simulink model "bergman"  (R2021a)
settings: Solver=FixedStepAuto  StartTime=0.0  StopTime=1440  FixedStep=Ts  RelTol=1e-3
values from neighbouring files (symbols this model uses):
  Ag = 0.95    [afterGA.m]    (also in identik.m; lakaka.m; surove.m)
  Gb = 153    [afterGA.m]    (also in bergmanGA.m = glucose(1); cv3.m = glucose(1); cv3a.m = glucose(1); cv4_bergman.m)
  Ib = 12.3165    [afterGA.m]    (also in bergmanGA.m = insuline(1); cv3.m = insuline(1); cv3a.m = insuline(1); cv4.m)
  kI = 0.1645    [afterGA.m]    (also in cv4.m = Best(2); cv4GA.m = Best(2); cv4_bergman.m; cv4_bergmanGA.m)
  p2 = 0.0106    [afterGA.m]    (also in cv3.m = 0.032736; cv3a.m = 0.063098; cv4_bergman.m = Best(2) / 10; cv4_bergmanGA.m = Best(2) / 10)
  S1b = 1.2528e4    (= 12528)    [afterGA.m]    (also in cv4.m; cv4GA.m; cv4_bergman.m; cv4_bergmanGA.m)
  S2b = S1b    (= 12528)    [afterGA.m]    (also in cv4.m; cv4GA.m; cv4_bergman.m; cv4_bergmanGA.m)
  Sg = 0.032    [afterGA.m]    (also in cv3.m = 0.030031; cv3a.m = 3.3574e-10; cv4_bergman.m = 0; cv4_bergmanGA.m = 0)
  Si = 0.00159    [afterGA.m]    (also in cv3.m = 1.0278e-13; cv3a.m = 0.00089844; cv4_bergman.m = Best(1) / 10; cv4_bergmanGA.m = Best(1) / 10)
  Td = 33.474    [afterGA.m]    (also in identified.mat = 40.284; identified1.mat = 33.5; lakaka.m; surove.m)
  TI = 44.55    [afterGA.m]    (also in cv4.m = Best(1); cv4GA.m = Best(1); cv4_bergman.m; cv4_bergmanGA.m)
  Vg = 1.467    [afterGA.m]    (also in cv4_bergman.m; cv4_bergmanGA.m; identik.m; lakaka.m)
  VI = 138.8    [afterGA.m]    (also in cv4.m = Best(3); cv4GA.m = Best(3); cv4_bergman.m; cv4_bergmanGA.m)
settings Model: Creator=marko  LastModifiedBy=marko

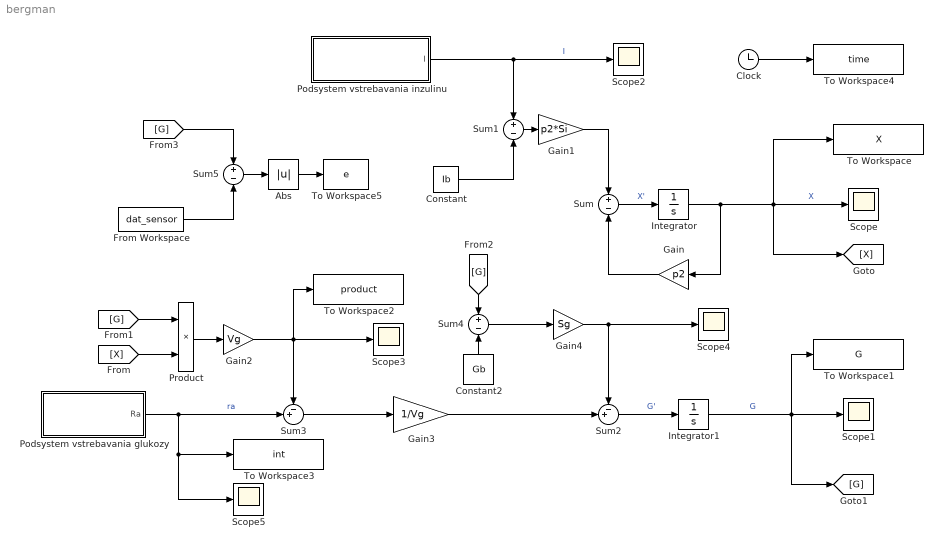
== system bergman ==
  Abs : Abs
  Clock : Clock
  Constant : Constant  Value=Ib
  Constant2 : Constant  Value=Gb
  From Workspace : FromWorkspace  VariableName=dat_sensor  Interpolate=off  OutputAfterFinalValue=Holding final value
  Gain : Gain  Gain=p2
  Gain1 : Gain  Gain=p2*Si
  Gain2 : Gain  Gain=Vg
  Gain3 : Gain  Gain=1/Vg
  Gain4 : Gain  Gain=Sg
  Integrator : Integrator
  Integrator1 : Integrator  InitialCondition=Gb
  Podsystem vstrebavania glukozy : Subsystem
  Podsystem vstrebavania inzulinu : Subsystem
  Product : Product
  Scope{,1..5} (6 alike) : Scope
  Sum{,1,4..5} (4 alike) : Sum  Inputs=+|-
  Sum2 : Sum  Inputs=-+|
  Sum3 : Sum  Inputs=-+|
  To Workspace : ToWorkspace  VariableName=X  SampleTime=-1
  To Workspace1 : ToWorkspace  VariableName=G  SampleTime=-1
  To Workspace2 : ToWorkspace  VariableName=product  SampleTime=-1
  To Workspace3 : ToWorkspace  VariableName=int  SampleTime=-1
  To Workspace4 : ToWorkspace  VariableName=time  SampleTime=-1
  To Workspace5 : ToWorkspace  VariableName=e  SampleTime=-1
  wires:
  Integrator/1 -> To Workspace/1, [X], Scope/1, Gain/1  "X"
  Gain/1 -> Sum/2
  Sum/1 -> Integrator/1  "X'"
  Constant/1 -> Sum1/2
  Sum1/1 -> Gain1/1
  Gain1/1 -> Sum/1
  Integrator1/1 -> Scope1/1, [G], To Workspace1/1  "G"
  Sum2/1 -> Integrator1/1  "G'"
  Podsystem vstrebavania inzulinu/1(I) -> Sum1/1, Scope2/1  "I"
  Podsystem vstrebavania glukozy/1(Ra) -> Scope5/1, To Workspace3/1, Sum3/2  "ra"
  Sum3/1 -> Gain3/1
  [G] -> Product/1
  [X] -> Product/2
  Product/1 -> Gain2/1
  Gain2/1 -> Scope3/1, To Workspace2/1, Sum3/1
  Gain3/1 -> Sum2/2
  [G] -> Sum4/1
  Constant2/1 -> Sum4/2
  Sum4/1 -> Gain4/1
  Gain4/1 -> Scope4/1, Sum2/1
  Clock/1 -> To Workspace4/1
  [G] -> Sum5/1
  From Workspace/1 -> Sum5/2
  Sum5/1 -> Abs/1
  Abs/1 -> To Workspace5/1

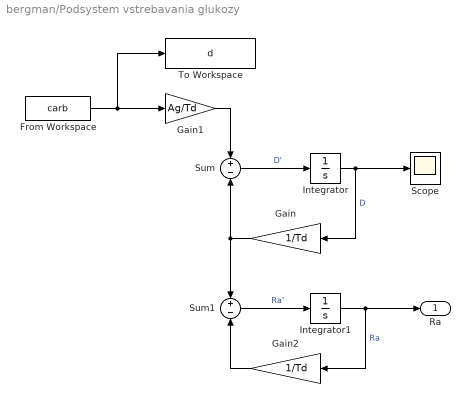
== system bergman/Podsystem vstrebavania glukozy ==
  From Workspace : FromWorkspace  VariableName=carb  Interpolate=off  OutputAfterFinalValue=Setting to zero
  Gain : Gain  Gain=1/Td
  Gain1 : Gain  Gain=Ag/Td
  Gain2 : Gain  Gain=1/Td
  Integrator : Integrator
  Integrator1 : Integrator
  Scope : Scope
  Sum : Sum  Inputs=+|-
  Sum1 : Sum  Inputs=+|-
  To Workspace : ToWorkspace  VariableName=d  SampleTime=-1
  Ra : Outport
  wires:
  Integrator1/1 -> Gain2/1, Ra/1  "Ra"
  Integrator/1 -> Scope/1, Gain/1  "D"
  Gain/1 -> Sum1/1, Sum/2
  Sum/1 -> Integrator/1  "D'"
  Gain1/1 -> Sum/1
  Sum1/1 -> Integrator1/1  "Ra'"
  Gain2/1 -> Sum1/2
  From Workspace/1 -> To Workspace/1, Gain1/1

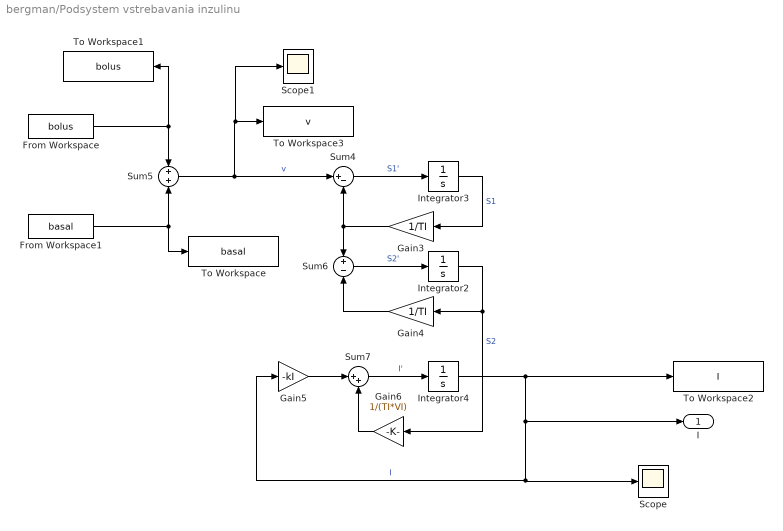
== system bergman/Podsystem vstrebavania inzulinu ==
  From Workspace : FromWorkspace  VariableName=bolus  Interpolate=off  OutputAfterFinalValue=Setting to zero
  From Workspace1 : FromWorkspace  VariableName=basal  Interpolate=off  OutputAfterFinalValue=Setting to zero
  Gain3 : Gain  Gain=1/TI
  Gain4 : Gain  Gain=1/TI
  Gain5 : Gain  Gain=-kI
  Gain6 : Gain  Gain=1/(TI*VI)
  Integrator2 : Integrator  InitialCondition=S2b
  Integrator3 : Integrator  InitialCondition=S1b
  Integrator4 : Integrator  InitialCondition=Ib
  Scope : Scope
  Scope1 : Scope
  Sum4 : Sum  Inputs=|+-
  Sum5 : Sum  Inputs=+|+
  Sum6 : Sum  Inputs=+|-
  Sum7 : Sum  Inputs=|++
  To Workspace : ToWorkspace  VariableName=basal  SaveFormat=Timeseries  SampleTime=-1
  To Workspace1 : ToWorkspace  VariableName=bolus  SaveFormat=Timeseries  SampleTime=-1
  To Workspace2 : ToWorkspace  VariableName=I  SampleTime=-1
  To Workspace3 : ToWorkspace  VariableName=v  SampleTime=-1
  I : Outport  VectorParamsAs1DForOutWhenUnconnected=off
  wires:
  Integrator4/1 -> I/1, Scope/1, Gain5/1, To Workspace2/1  "I"
  Gain3/1 -> Sum4/2, Sum6/1
  Gain4/1 -> Sum6/2
  Sum4/1 -> Integrator3/1  "S1'"
  Gain5/1 -> Sum7/1
  Sum7/1 -> Integrator4/1  "I'"
  Integrator2/1 -> Gain6/1, Gain4/1  "S2"
  Sum6/1 -> Integrator2/1  "S2'"
  Gain6/1 -> Sum7/2
  Sum5/1 -> Scope1/1, To Workspace3/1, Sum4/1  "v"
  Integrator3/1 -> Gain3/1  "S1"
  From Workspace/1 -> To Workspace1/1, Sum5/1
  From Workspace1/1 -> To Workspace/1, Sum5/2
